simulink model "ES300A_SinVltgGenn"  (R2013b)
settings: Solver=FixedStepDiscrete  StartTime=0.0  StopTime=5  RelTol=1e-3
values from neighbouring files (symbols this model uses):
  ELECGLBPRM_PWMPERDMAX_NANOSEC_U32 = DataDict.ConfigParam    [ES300A_SinVltgGenn_DataDict.m]
  ELECGLBPRM_PWMPERDMIN_NANOSEC_U32 = DataDict.ConfigParam    [ES300A_SinVltgGenn_DataDict.m]
  SINVLTGGENN120DEG_MOTREVELEC_F32 = DataDict.Constant    [ES300A_SinVltgGenn_DataDict.m]
  SINVLTGGENN240DEG_MOTREVELEC_F32 = DataDict.Constant    [ES300A_SinVltgGenn_DataDict.m]
  SINVLTGGENN60DEG_MOTREVELEC_F32 = DataDict.Constant    [ES300A_SinVltgGenn_DataDict.m]
  SINVLTGGENNCMUOFFSTBLX_ULS_F32 = DataDict.Constant    [ES300A_SinVltgGenn_DataDict.m]
  SINVLTGGENNCMUOFFSTBLY_NANOSEC_F32 = DataDict.Constant    [ES300A_SinVltgGenn_DataDict.m]
  SinVltgGennDthrLpFilCoeff = DataDict.Calibration    [ES300A_SinVltgGenn_DataDict.m]
  SINVLTGGENNPHAONTIMAXLIM_NANOSEC_U32 = DataDict.Constant    [ES300A_SinVltgGenn_DataDict.m]
  SINVLTGGENNPHAONTISUMMAXLIM_NANOSEC_U32 = DataDict.Constant    [ES300A_SinVltgGenn_DataDict.m]
  SINVLTGGENNPHATOGNDTBL_CNT_U16 = DataDict.Constant    [ES300A_SinVltgGenn_DataDict.m]
  SINVLTGGENNPHATOGNDTBLSIZE_CNT_U16 = DataDict.Constant    [ES300A_SinVltgGenn_DataDict.m]
  SINVLTGGENNSEEDINI_ULS_F32 = DataDict.Constant    [ES300A_SinVltgGenn_DataDict.m]
  SINVLTGGENNSEEDMPLR_ULS_U08 = DataDict.Constant    [ES300A_SinVltgGenn_DataDict.m]
  SINVLTGGENNSEEDOFFS_ULS_F32 = DataDict.Constant    [ES300A_SinVltgGenn_DataDict.m]
  SINVLTGGENNZERODEG_MOTREVELEC_F32 = DataDict.Constant    [ES300A_SinVltgGenn_DataDict.m]
libraries: simulink x10, FixdToFloat x2
(part 2 of 2)

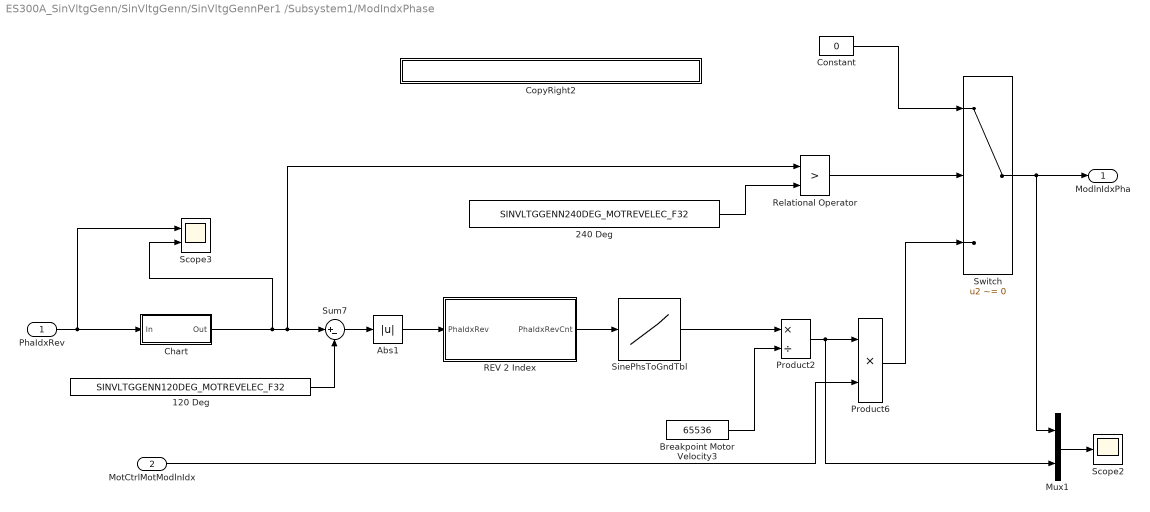
== system ES300A_SinVltgGenn/SinVltgGenn/SinVltgGennPer1 /Subsystem1/ModIndxPhase ==
  "PhaIdxRev " : Inport
  MotCtrlMotModlnIdx : Inport  Port=2
  120 Deg : Constant  Value=SINVLTGGENN120DEG_MOTREVELEC_F32
  240 Deg : Constant  Value=SINVLTGGENN240DEG_MOTREVELEC_F32
  Abs1 : Abs
  Breakpoint Motor Velocity3 : Constant  Value=65536  OutDataTypeStr=single
  Chart : Stateflow chart  TreatAsAtomicUnit=on
  Constant : Constant  Value=0  OutDataTypeStr=single
  CopyRight2 : Subsystem  Description=|  mask(Copyright Information){none=on}
      | Copyright info block.                                               
      |                                                                     
      | Place copyright information at the top of every subsystem in design.
      mask prompts: none "No parameters"
      mask help: Place copyright information at the top of every subsystem in design.
      mask Display:
      | NxtrConf = 'Nexteer Confidential';
      | 
      | sys = bdroot; %handle for the current model ("system")
      | first = get_param(sys,'Created');
      | first = first(end-3:end);  %year is last four digits
      | 
      | last = get_param(sys,'LastModifiedDate');
      | if isempty(last)
      |     last = datestr(now,'yyyy');
      | else
      |     last = last(end-3:end);
      | end
      | 
      | if strcmp(first,last)
      |     fprintf('%s -- Copyright %s Nexteer',NxtrConf,first)
      | else
      |     fprintf('%s -- %s%s- %s Nexteer',NxtrConf,char(169),first,last)
      | end
  Mux1 : Mux  Inputs=2
  Product2 : Product  Inputs=*/  RndMeth=Zero
  Product6 : Product  RndMeth=Zero
  REV 2 Index : Subsystem
  Relational Operator : RelationalOperator  Operator=>  OutDataTypeStr=boolean
  Scope2 : Scope
      settings: YMin=0  YMax=1  SaveName=ScopeData5
  Scope3 : Scope  NumInputPorts=2
      settings: TimeRange=20  YMin=0~0  YMax=2.25~1  SaveName=ScopeData10
  SinePhsToGndTbl : Lookup  InputValues=0:length(SINVLTGGENNPHATOGNDTBL_CNT_U16)-1  Table=SINVLTGGENNPHATOGNDTBL_CNT_U16  LookUpMeth=Interpolation-Use End Values
      settings: AttributesFormatString=%<Table>\n%<InputValues>
  Sum7 : Sum  Inputs=|+-
  Switch : Switch  Criteria=u2 ~= 0
  ModlnIdxPha : Outport
  wires:
  "PhaIdxRev "/1 -> Scope3/1, Chart/1(In)
  Abs1/1 -> REV 2 Index/1("PhaIdxRev ")
  REV 2 Index/1(PhaIdxRevCnt) -> SinePhsToGndTbl/1
  Product2/1 -> Mux1/2, Product6/1
  Relational Operator/1 -> Switch/2
  Constant/1 -> Switch/1
  Product6/1 -> Switch/3
  Sum7/1 -> Abs1/1
  SinePhsToGndTbl/1 -> Product2/1
  Breakpoint Motor Velocity3/1 -> Product2/2
  Chart/1(Out) -> Scope3/2, Sum7/1, Relational Operator/1
  120 Deg/1 -> Sum7/2
  MotCtrlMotModlnIdx/1 -> Product6/2
  240 Deg/1 -> Relational Operator/2
  Mux1/1 -> Scope2/1
  Switch/1 -> Mux1/1, ModlnIdxPha/1

== system ES300A_SinVltgGenn/SinVltgGenn/SinVltgGennPer1 /Subsystem2/CopyRight2 ==

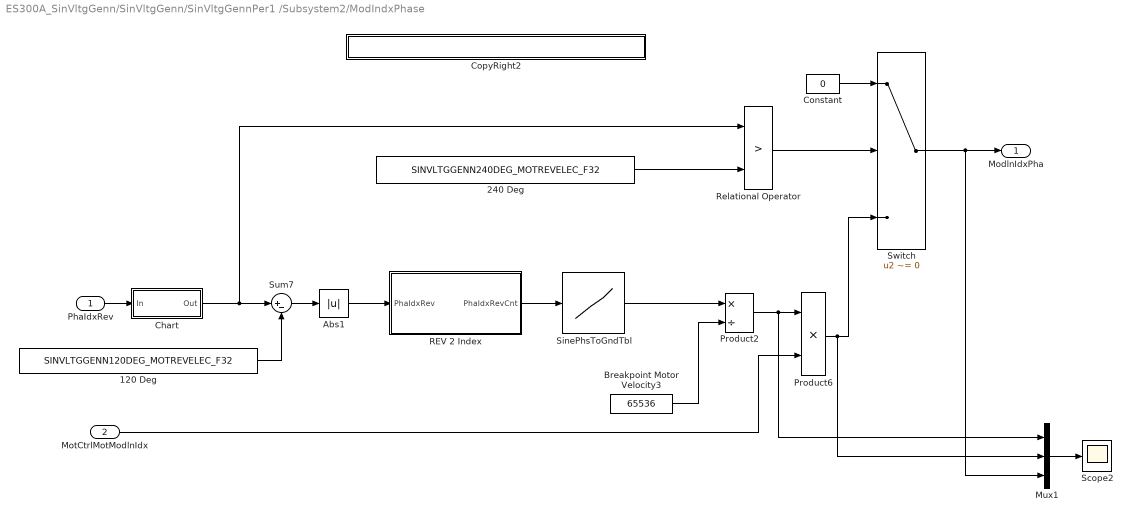
== system ES300A_SinVltgGenn/SinVltgGenn/SinVltgGennPer1 /Subsystem2/ModIndxPhase ==
  "PhaIdxRev " : Inport
  MotCtrlMotModlnIdx : Inport  Port=2
  120 Deg : Constant  Value=SINVLTGGENN120DEG_MOTREVELEC_F32
  240 Deg : Constant  Value=SINVLTGGENN240DEG_MOTREVELEC_F32
  Abs1 : Abs
  Breakpoint Motor Velocity3 : Constant  Value=65536  OutDataTypeStr=single
  Chart : Stateflow chart  TreatAsAtomicUnit=on
  Constant : Constant  Value=0  OutDataTypeStr=single
  CopyRight2 : Subsystem  Description=|  mask(Copyright Information){none=on}
      | Copyright info block.                                               
      |                                                                     
      | Place copyright information at the top of every subsystem in design.
      mask prompts: none "No parameters"
      mask help: Place copyright information at the top of every subsystem in design.
      mask Display:
      | NxtrConf = 'Nexteer Confidential';
      | 
      | sys = bdroot; %handle for the current model ("system")
      | first = get_param(sys,'Created');
      | first = first(end-3:end);  %year is last four digits
      | 
      | last = get_param(sys,'LastModifiedDate');
      | if isempty(last)
      |     last = datestr(now,'yyyy');
      | else
      |     last = last(end-3:end);
      | end
      | 
      | if strcmp(first,last)
      |     fprintf('%s -- Copyright %s Nexteer',NxtrConf,first)
      | else
      |     fprintf('%s -- %s%s- %s Nexteer',NxtrConf,char(169),first,last)
      | end
  Mux1 : Mux  Inputs=3
  Product2 : Product  Inputs=*/  RndMeth=Zero
  Product6 : Product  RndMeth=Zero
  REV 2 Index : Subsystem
  Relational Operator : RelationalOperator  Operator=>  OutDataTypeStr=boolean
  Scope2 : Scope
      settings: YMin=2500  YMax=40000  SaveName=ScopeData5
  SinePhsToGndTbl : Lookup  InputValues=0:length(SINVLTGGENNPHATOGNDTBL_CNT_U16)-1  Table=SINVLTGGENNPHATOGNDTBL_CNT_U16  LookUpMeth=Interpolation-Use End Values
      settings: AttributesFormatString=%<Table>\n%<InputValues>
  Sum7 : Sum  Inputs=|+-
  Switch : Switch  Criteria=u2 ~= 0
  ModlnIdxPha : Outport
  wires:
  "PhaIdxRev "/1 -> Chart/1(In)
  Abs1/1 -> REV 2 Index/1("PhaIdxRev ")
  REV 2 Index/1(PhaIdxRevCnt) -> SinePhsToGndTbl/1
  Product2/1 -> Mux1/1, Product6/1
  Switch/1 -> Mux1/3, ModlnIdxPha/1
  Relational Operator/1 -> Switch/2
  Constant/1 -> Switch/1
  Product6/1 -> Mux1/2, Switch/3
  Sum7/1 -> Abs1/1
  SinePhsToGndTbl/1 -> Product2/1
  Breakpoint Motor Velocity3/1 -> Product2/2
  Chart/1(Out) -> Sum7/1, Relational Operator/1
  120 Deg/1 -> Sum7/2
  MotCtrlMotModlnIdx/1 -> Product6/2
  240 Deg/1 -> Relational Operator/2
  Mux1/1 -> Scope2/1

== system ES300A_SinVltgGenn/SinVltgGenn/SinVltgGennPer1 /Subsystem3/CopyRight2 ==

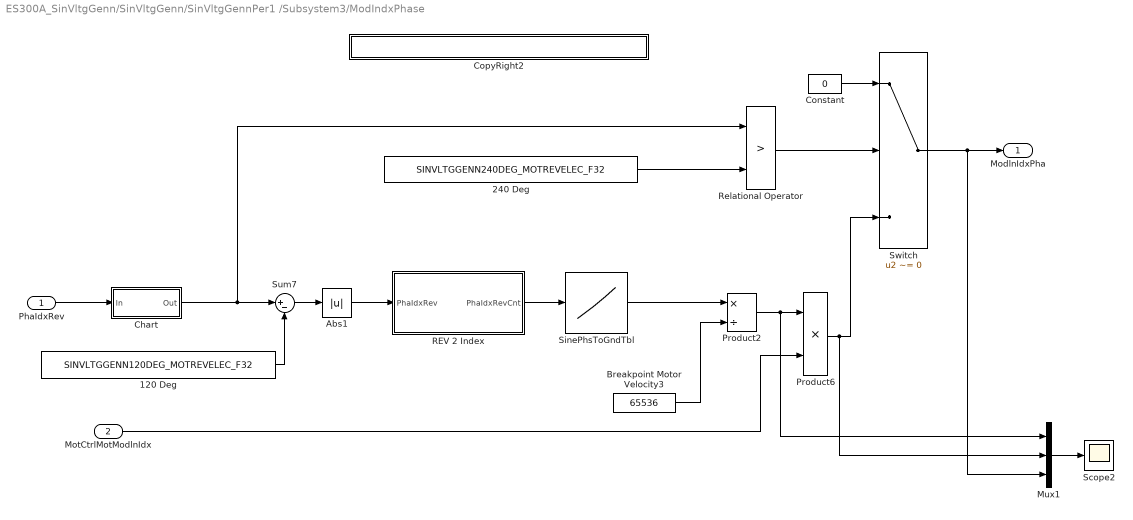
== system ES300A_SinVltgGenn/SinVltgGenn/SinVltgGennPer1 /Subsystem3/ModIndxPhase ==
  "PhaIdxRev " : Inport  OutDataTypeStr=single
  MotCtrlMotModlnIdx : Inport  Port=2
  120 Deg : Constant  Value=SINVLTGGENN120DEG_MOTREVELEC_F32
  240 Deg : Constant  Value=SINVLTGGENN240DEG_MOTREVELEC_F32
  Abs1 : Abs
  Breakpoint Motor Velocity3 : Constant  Value=65536  OutDataTypeStr=single
  Chart : Stateflow chart  TreatAsAtomicUnit=on
  Constant : Constant  Value=0  OutDataTypeStr=single
  CopyRight2 : Subsystem  Description=|  mask(Copyright Information){none=on}
      | Copyright info block.                                               
      |                                                                     
      | Place copyright information at the top of every subsystem in design.
      mask prompts: none "No parameters"
      mask help: Place copyright information at the top of every subsystem in design.
      mask Display:
      | NxtrConf = 'Nexteer Confidential';
      | 
      | sys = bdroot; %handle for the current model ("system")
      | first = get_param(sys,'Created');
      | first = first(end-3:end);  %year is last four digits
      | 
      | last = get_param(sys,'LastModifiedDate');
      | if isempty(last)
      |     last = datestr(now,'yyyy');
      | else
      |     last = last(end-3:end);
      | end
      | 
      | if strcmp(first,last)
      |     fprintf('%s -- Copyright %s Nexteer',NxtrConf,first)
      | else
      |     fprintf('%s -- %s%s- %s Nexteer',NxtrConf,char(169),first,last)
      | end
  Mux1 : Mux  Inputs=3
  Product2 : Product  Inputs=*/  RndMeth=Zero
  Product6 : Product  RndMeth=Zero
  REV 2 Index : Subsystem
  Relational Operator : RelationalOperator  Operator=>  OutDataTypeStr=boolean
  Scope2 : Scope
      settings: YMin=2500  YMax=40000  SaveName=ScopeData5
  SinePhsToGndTbl : Lookup  InputValues=0:length(SINVLTGGENNPHATOGNDTBL_CNT_U16)-1  Table=SINVLTGGENNPHATOGNDTBL_CNT_U16  LookUpMeth=Interpolation-Use End Values
      settings: AttributesFormatString=%<Table>\n%<InputValues>
  Sum7 : Sum  Inputs=|+-
  Switch : Switch  Criteria=u2 ~= 0
  ModlnIdxPha : Outport
  wires:
  "PhaIdxRev "/1 -> Chart/1(In)
  Abs1/1 -> REV 2 Index/1("PhaIdxRev ")
  REV 2 Index/1(PhaIdxRevCnt) -> SinePhsToGndTbl/1
  Product2/1 -> Mux1/1, Product6/1
  Switch/1 -> Mux1/3, ModlnIdxPha/1
  Relational Operator/1 -> Switch/2
  Constant/1 -> Switch/1
  Product6/1 -> Mux1/2, Switch/3
  Sum7/1 -> Abs1/1
  SinePhsToGndTbl/1 -> Product2/1
  Breakpoint Motor Velocity3/1 -> Product2/2
  Chart/1(Out) -> Sum7/1, Relational Operator/1
  120 Deg/1 -> Sum7/2
  MotCtrlMotModlnIdx/1 -> Product6/2
  240 Deg/1 -> Relational Operator/2
  Mux1/1 -> Scope2/1

== system ES300A_SinVltgGenn/SinVltgGenn/SinVltgGennPer1 /PWMPeriodDither_U16 /Filter1/CopyRight2 ==

== system ES300A_SinVltgGenn/SinVltgGenn/SinVltgGennPer1 /PWMPeriodDither_U16 /Filter2/CopyRight2 ==

== system ES300A_SinVltgGenn/SinVltgGenn/SinVltgGennPer1 /PWMPeriodDither_U16 /RandomNumberGenerator/CopyRight2 ==

== system ES300A_SinVltgGenn/SinVltgGenn/SinVltgGennPer1 /Subsystem1/ModIndxPhase/CopyRight2 ==

== system ES300A_SinVltgGenn/SinVltgGenn/SinVltgGennPer1 /Subsystem1/ModIndxPhase/REV 2 Index ==
  "PhaIdxRev " : Inport
  120 Deg : Constant  Value=SINVLTGGENN120DEG_MOTREVELEC_F32
  2049 : Constant  Value=SINVLTGGENNPHATOGNDTBLSIZE_CNT_U16
  Breakpoint Motor Velocity2 : Constant  Value=0.5  OutDataTypeStr=single
  CopyRight2 : Subsystem  Description=|  mask(Copyright Information){none=on}
      | Copyright info block.                                               
      |                                                                     
      | Place copyright information at the top of every subsystem in design.
      mask prompts: none "No parameters"
      mask help: Place copyright information at the top of every subsystem in design.
      mask Display:
      | NxtrConf = 'Nexteer Confidential';
      | 
      | sys = bdroot; %handle for the current model ("system")
      | first = get_param(sys,'Created');
      | first = first(end-3:end);  %year is last four digits
      | 
      | last = get_param(sys,'LastModifiedDate');
      | if isempty(last)
      |     last = datestr(now,'yyyy');
      | else
      |     last = last(end-3:end);
      | end
      | 
      | if strcmp(first,last)
      |     fprintf('%s -- Copyright %s Nexteer',NxtrConf,first)
      | else
      |     fprintf('%s -- %s%s- %s Nexteer',NxtrConf,char(169),first,last)
      | end
  Divide : Product  Inputs=*/
  Product1 : Product  RndMeth=Zero
  Rounding Function : Rounding
  Sum1 : Sum  Inputs=|++
  Sum2 : Sum  Inputs=+-
  constant : Constant  OutDataTypeStr=single
  PhaIdxRevCnt : Outport
  wires:
  "PhaIdxRev "/1 -> Product1/1
  Product1/1 -> Sum1/1
  Breakpoint Motor Velocity2/1 -> Sum1/2
  Sum1/1 -> Rounding Function/1
  Rounding Function/1 -> PhaIdxRevCnt/1
  120 Deg/1 -> Divide/2
  2049/1 -> Sum2/1
  constant/1 -> Sum2/2
  Sum2/1 -> Divide/1
  Divide/1 -> Product1/2

== system ES300A_SinVltgGenn/SinVltgGenn/SinVltgGennPer1 /Subsystem2/ModIndxPhase/CopyRight2 ==

== system ES300A_SinVltgGenn/SinVltgGenn/SinVltgGennPer1 /Subsystem2/ModIndxPhase/REV 2 Index ==
  "PhaIdxRev " : Inport
  120 Deg : Constant  Value=SINVLTGGENN120DEG_MOTREVELEC_F32
  2049 : Constant  Value=SINVLTGGENNPHATOGNDTBLSIZE_CNT_U16
  Breakpoint Motor Velocity2 : Constant  Value=0.5  OutDataTypeStr=single
  CopyRight2 : Subsystem  Description=|  mask(Copyright Information){none=on}
      | Copyright info block.                                               
      |                                                                     
      | Place copyright information at the top of every subsystem in design.
      mask prompts: none "No parameters"
      mask help: Place copyright information at the top of every subsystem in design.
      mask Display:
      | NxtrConf = 'Nexteer Confidential';
      | 
      | sys = bdroot; %handle for the current model ("system")
      | first = get_param(sys,'Created');
      | first = first(end-3:end);  %year is last four digits
      | 
      | last = get_param(sys,'LastModifiedDate');
      | if isempty(last)
      |     last = datestr(now,'yyyy');
      | else
      |     last = last(end-3:end);
      | end
      | 
      | if strcmp(first,last)
      |     fprintf('%s -- Copyright %s Nexteer',NxtrConf,first)
      | else
      |     fprintf('%s -- %s%s- %s Nexteer',NxtrConf,char(169),first,last)
      | end
  Divide : Product  Inputs=*/
  Product1 : Product  RndMeth=Zero
  Rounding Function : Rounding
  Sum1 : Sum  Inputs=|++
  Sum2 : Sum  Inputs=+-
  constant : Constant  OutDataTypeStr=single
  PhaIdxRevCnt : Outport
  wires:
  "PhaIdxRev "/1 -> Product1/1
  Product1/1 -> Sum1/1
  Breakpoint Motor Velocity2/1 -> Sum1/2
  Sum1/1 -> Rounding Function/1
  Rounding Function/1 -> PhaIdxRevCnt/1
  120 Deg/1 -> Divide/2
  2049/1 -> Sum2/1
  constant/1 -> Sum2/2
  Sum2/1 -> Divide/1
  Divide/1 -> Product1/2

== system ES300A_SinVltgGenn/SinVltgGenn/SinVltgGennPer1 /Subsystem3/ModIndxPhase/CopyRight2 ==

== system ES300A_SinVltgGenn/SinVltgGenn/SinVltgGennPer1 /Subsystem3/ModIndxPhase/REV 2 Index ==
  "PhaIdxRev " : Inport
  120 Deg : Constant  Value=SINVLTGGENN120DEG_MOTREVELEC_F32
  2049 : Constant  Value=SINVLTGGENNPHATOGNDTBLSIZE_CNT_U16
  Breakpoint Motor Velocity2 : Constant  Value=0.5  OutDataTypeStr=single
  CopyRight2 : Subsystem  Description=|  mask(Copyright Information){none=on}
      | Copyright info block.                                               
      |                                                                     
      | Place copyright information at the top of every subsystem in design.
      mask prompts: none "No parameters"
      mask help: Place copyright information at the top of every subsystem in design.
      mask Display:
      | NxtrConf = 'Nexteer Confidential';
      | 
      | sys = bdroot; %handle for the current model ("system")
      | first = get_param(sys,'Created');
      | first = first(end-3:end);  %year is last four digits
      | 
      | last = get_param(sys,'LastModifiedDate');
      | if isempty(last)
      |     last = datestr(now,'yyyy');
      | else
      |     last = last(end-3:end);
      | end
      | 
      | if strcmp(first,last)
      |     fprintf('%s -- Copyright %s Nexteer',NxtrConf,first)
      | else
      |     fprintf('%s -- %s%s- %s Nexteer',NxtrConf,char(169),first,last)
      | end
  Divide : Product  Inputs=*/
  Product1 : Product  RndMeth=Zero
  Rounding Function : Rounding
  Sum1 : Sum  Inputs=|++
  Sum2 : Sum  Inputs=+-
  constant : Constant  OutDataTypeStr=single
  PhaIdxRevCnt : Outport
  wires:
  "PhaIdxRev "/1 -> Product1/1
  Product1/1 -> Sum1/1
  Breakpoint Motor Velocity2/1 -> Sum1/2
  Sum1/1 -> Rounding Function/1
  Rounding Function/1 -> PhaIdxRevCnt/1
  120 Deg/1 -> Divide/2
  2049/1 -> Sum2/1
  constant/1 -> Sum2/2
  Sum2/1 -> Divide/1
  Divide/1 -> Product1/2

== system ES300A_SinVltgGenn/SinVltgGenn/SinVltgGennPer1 /Subsystem1/ModIndxPhase/REV 2 Index/CopyRight2 ==

== system ES300A_SinVltgGenn/SinVltgGenn/SinVltgGennPer1 /Subsystem2/ModIndxPhase/REV 2 Index/CopyRight2 ==

== system ES300A_SinVltgGenn/SinVltgGenn/SinVltgGennPer1 /Subsystem3/ModIndxPhase/REV 2 Index/CopyRight2 ==

== stateflow chart ES300A_SinVltgGenn/SinVltgGenn/SinVltgGennPer1 /Subsystem1/ModIndxPhase/Chart ==
  (default) -> (junction 1) : {Out = In;}
  (junction 1) -> (junction 3) [order 2] : [Out < 0]
      | {Out = Out + 1;}
  (junction 1) -> (junction 4) [order 1] : [Out > 1]
      | {Out = Out - 1;}
  (junction 4) -> (junction 1)
  (junction 3) -> (junction 1)
  (junction 1) -> (junction 5) [order 3]
  data: In input; Out output single

== stateflow chart ES300A_SinVltgGenn/SinVltgGenn/SinVltgGennPer1 /Subsystem2/ModIndxPhase/Chart ==
  (default) -> (junction 1) : {Out = In;}
  (junction 1) -> (junction 3) [order 2] : [Out < 0]
      | {Out = Out + 1;}
  (junction 1) -> (junction 4) [order 1] : [Out > 1]
      | {Out = Out - 1;}
  (junction 4) -> (junction 1)
  (junction 3) -> (junction 1)
  (junction 1) -> (junction 5) [order 3]
  data: In input; Out output single

== stateflow chart ES300A_SinVltgGenn/SinVltgGenn/SinVltgGennPer1 /Subsystem3/ModIndxPhase/Chart ==
  (default) -> (junction 1) : {Out = In;}
  (junction 1) -> (junction 3) [order 2] : [Out < 0]
      | {Out = Out + 1;}
  (junction 1) -> (junction 4) [order 1] : [Out > 1]
      | {Out = Out - 1;}
  (junction 4) -> (junction 1)
  (junction 3) -> (junction 1)
  (junction 1) -> (junction 5) [order 3]
  data: In input; Out output single
